simulink library "lib_inverse_clarke_transform"  (R2023a)
settings: Solver=VariableStepAuto  StartTime=0.0  StopTime=10.0  RelTol=1e-3
settings Model: Creator=cav2ofo  LastModifiedBy=lenovo
settings OptimizationCC: ReuseModelBlockBuffer=off

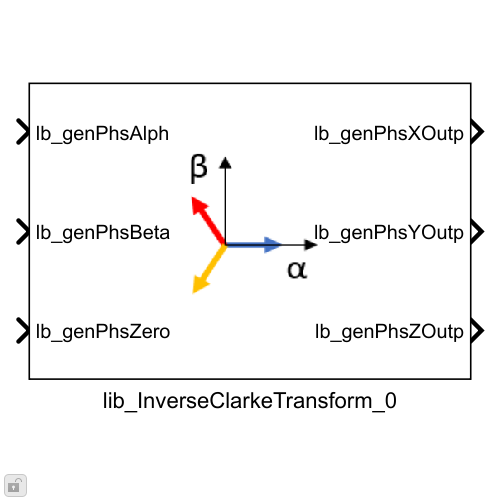
[thumbnail: Simulink's stored preview of the top-level diagram]
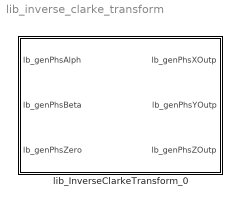
== system lib_inverse_clarke_transform ==
  lib_InverseClarkeTransform_0 : Subsystem  VariantControl=ClarkTransf_MIL_flo  mask{lb_parSymMot=off}
      mask prompts: lb_parSymMot "Asymmetric motor"
      mask DialogControl DescGroupVar Prompt: Inverse Clarke Transform
      mask DialogControl DescTextVar Prompt: VHIT Control Library
      mask DialogControl clarkeDesc Prompt: This block performs Inverse Clarke transform on the input signals. You can choose the computation logic either for symmetric or asymmetric motor type. For symmetric motor type the lb_genPhsZero is zero.
      mask DialogControl blockParam Prompt: Block Parameters
      mask DialogControl Control2 Prompt: By default the computation for symmetric motor is performed. Tick the following check box for asymmetric motor type.
      mask Display: image('ClarkTransf.png'); % Use "Edit Image" on toolstrip to change.

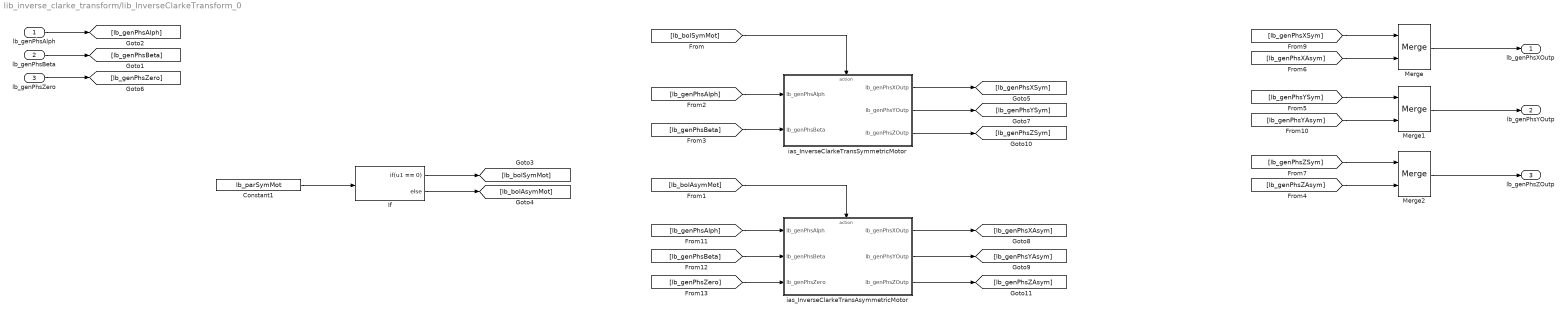
== system lib_inverse_clarke_transform/lib_InverseClarkeTransform_0 ==
  lb_genPhsAlph : Inport
  lb_genPhsBeta : Inport  Port=2
  lb_genPhsZero : Inport  Port=3
  Constant1 : Constant  Value=lb_parSymMot  OutDataTypeStr=boolean
  If : If  IfExpression=u1 == 0
  Merge : Merge
  Merge1 : Merge
  Merge2 : Merge
  ias_InverseClarkeTransAsymmetricMotor : Subsystem  TreatAsAtomicUnit=on
  ias_InverseClarkeTransSymmetricMotor : Subsystem  TreatAsAtomicUnit=on
  lb_genPhsXOutp : Outport  VectorParamsAs1DForOutWhenUnconnected=off
  lb_genPhsYOutp : Outport  Port=2  VectorParamsAs1DForOutWhenUnconnected=off
  lb_genPhsZOutp : Outport  Port=3  VectorParamsAs1DForOutWhenUnconnected=off
  wires:
  [lb_genPhsBeta] -> ias_InverseClarkeTransAsymmetricMotor/2(lb_genPhsBeta)
  If/1 -> [lb_bolSymMot]
  If/2 -> [lb_bolAsymMot]
  Merge2/1 -> lb_genPhsZOutp/1
  [lb_genPhsZSym] -> Merge2/1
  [lb_genPhsZAsym] -> Merge2/2
  ias_InverseClarkeTransAsymmetricMotor/3(lb_genPhsZOutp) -> [lb_genPhsZAsym]
  ias_InverseClarkeTransSymmetricMotor/3(lb_genPhsZOutp) -> [lb_genPhsZSym]
  [lb_genPhsZero] -> ias_InverseClarkeTransAsymmetricMotor/3(lb_genPhsZero)
  [lb_genPhsAlph] -> ias_InverseClarkeTransAsymmetricMotor/1(lb_genPhsAlph)
  lb_genPhsZero/1 -> [lb_genPhsZero]
  lb_genPhsBeta/1 -> [lb_genPhsBeta]
  lb_genPhsAlph/1 -> [lb_genPhsAlph]
  Merge/1 -> lb_genPhsXOutp/1
  Merge1/1 -> lb_genPhsYOutp/1
  [lb_genPhsYSym] -> Merge1/1
  [lb_genPhsYAsym] -> Merge1/2
  [lb_genPhsXAsym] -> Merge/2
  [lb_genPhsXSym] -> Merge/1
  ias_InverseClarkeTransAsymmetricMotor/2(lb_genPhsYOutp) -> [lb_genPhsYAsym]
  ias_InverseClarkeTransAsymmetricMotor/1(lb_genPhsXOutp) -> [lb_genPhsXAsym]
  ias_InverseClarkeTransSymmetricMotor/2(lb_genPhsYOutp) -> [lb_genPhsYSym]
  ias_InverseClarkeTransSymmetricMotor/1(lb_genPhsXOutp) -> [lb_genPhsXSym]
  [lb_genPhsBeta] -> ias_InverseClarkeTransSymmetricMotor/2(lb_genPhsBeta)
  [lb_genPhsAlph] -> ias_InverseClarkeTransSymmetricMotor/1(lb_genPhsAlph)
  [lb_bolAsymMot] -> ias_InverseClarkeTransAsymmetricMotor/Action
  [lb_bolSymMot] -> ias_InverseClarkeTransSymmetricMotor/Action
  Constant1/1 -> If/1

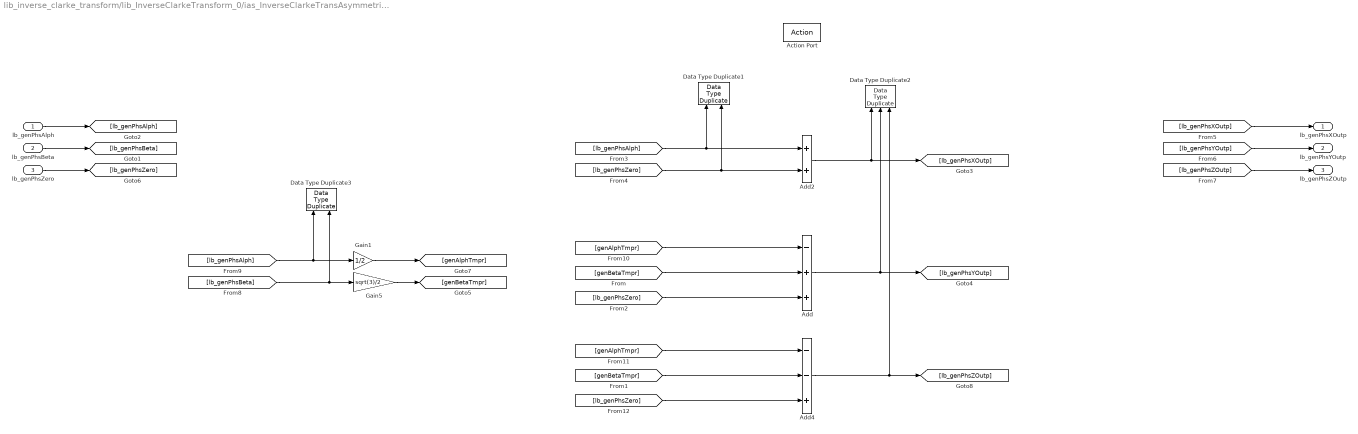
== system lib_inverse_clarke_transform/lib_InverseClarkeTransform_0/ias_InverseClarkeTransAsymmetricMotor ==
  lb_genPhsAlph : Inport
  lb_genPhsBeta : Inport  Port=2
  lb_genPhsZero : Inport  Port=3
  Action Port : ActionPort
  Add : Sum  Inputs=-++  OutDataTypeStr=Inherit: Inherit via back propagation  InputSameDT=on  SaturateOnIntegerOverflow=on
  Add2 : Sum  OutDataTypeStr=Inherit: Inherit via back propagation  InputSameDT=on  SaturateOnIntegerOverflow=on
  Add4 : Sum  Inputs=--+  OutDataTypeStr=Inherit: Inherit via back propagation  InputSameDT=on  SaturateOnIntegerOverflow=on
  Data Type Duplicate1 : DataTypeDuplicate
  Data Type Duplicate2 : DataTypeDuplicate  NumInputPorts=3
  Data Type Duplicate3 : DataTypeDuplicate
  Gain1 : Gain  Gain=1/2  OutDataTypeStr=Inherit: Inherit via back propagation
  Gain5 : Gain  Gain=sqrt(3)/2  ParamDataTypeStr=Inherit: Inherit from 'Gain'  OutDataTypeStr=Inherit: Inherit via back propagation
  lb_genPhsXOutp : Outport  VectorParamsAs1DForOutWhenUnconnected=off
  lb_genPhsYOutp : Outport  Port=2  VectorParamsAs1DForOutWhenUnconnected=off
  lb_genPhsZOutp : Outport  Port=3  VectorParamsAs1DForOutWhenUnconnected=off
  wires:
  [lb_genPhsZero] -> Add4/3
  [genBetaTmpr] -> Add4/2
  Add4/1 -> Data Type Duplicate2/3, [lb_genPhsZOutp]
  [genAlphTmpr] -> Add4/1
  Gain5/1 -> [genBetaTmpr]
  [lb_genPhsAlph] -> Gain1/1, Data Type Duplicate3/1
  [lb_genPhsBeta] -> Gain5/1, Data Type Duplicate3/2
  Gain1/1 -> [genAlphTmpr]
  [genAlphTmpr] -> Add/1
  [lb_genPhsZOutp] -> lb_genPhsZOutp/1
  [lb_genPhsYOutp] -> lb_genPhsYOutp/1
  [lb_genPhsXOutp] -> lb_genPhsXOutp/1
  lb_genPhsAlph/1 -> [lb_genPhsAlph]
  lb_genPhsBeta/1 -> [lb_genPhsBeta]
  lb_genPhsZero/1 -> [lb_genPhsZero]
  [lb_genPhsAlph] -> Add2/1, Data Type Duplicate1/1
  [genBetaTmpr] -> Add/2
  [lb_genPhsZero] -> Add2/2, Data Type Duplicate1/2
  [lb_genPhsZero] -> Add/3
  Add2/1 -> [lb_genPhsXOutp], Data Type Duplicate2/1
  Add/1 -> [lb_genPhsYOutp], Data Type Duplicate2/2

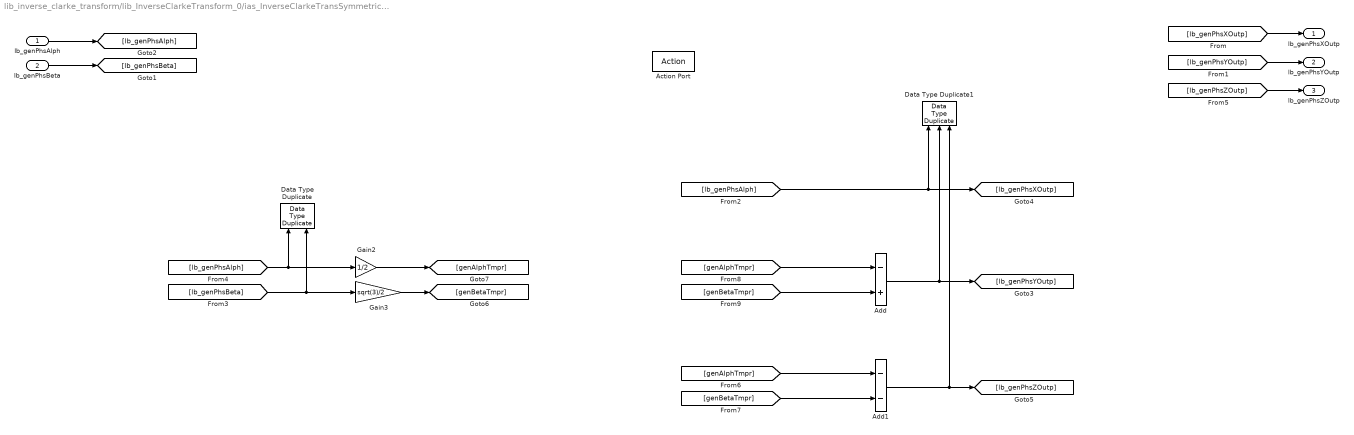
== system lib_inverse_clarke_transform/lib_InverseClarkeTransform_0/ias_InverseClarkeTransSymmetricMotor ==
  lb_genPhsAlph : Inport
  lb_genPhsBeta : Inport  Port=2
  Action Port : ActionPort
  Add : Sum  Inputs=-+  OutDataTypeStr=Inherit: Inherit via back propagation
  Add1 : Sum  Inputs=--  OutDataTypeStr=Inherit: Inherit via back propagation
  Data Type Duplicate : DataTypeDuplicate
  Data Type Duplicate1 : DataTypeDuplicate  NumInputPorts=3
  Gain2 : Gain  Gain=1/2  OutDataTypeStr=Inherit: Inherit via back propagation
  Gain3 : Gain  Gain=sqrt(3)/2  ParamDataTypeStr=Inherit: Inherit from 'Gain'  OutDataTypeStr=Inherit: Inherit via back propagation
  lb_genPhsXOutp : Outport  VectorParamsAs1DForOutWhenUnconnected=off
  lb_genPhsYOutp : Outport  Port=2  VectorParamsAs1DForOutWhenUnconnected=off
  lb_genPhsZOutp : Outport  Port=3  VectorParamsAs1DForOutWhenUnconnected=off
  wires:
  [genAlphTmpr] -> Add/1
  [genBetaTmpr] -> Add/2
  Add1/1 -> Data Type Duplicate1/3, [lb_genPhsZOutp]
  [genBetaTmpr] -> Add1/2
  [genAlphTmpr] -> Add1/1
  Gain2/1 -> [genAlphTmpr]
  [lb_genPhsZOutp] -> lb_genPhsZOutp/1
  [lb_genPhsAlph] -> [lb_genPhsXOutp], Data Type Duplicate1/1
  [lb_genPhsAlph] -> Data Type Duplicate/1, Gain2/1
  Gain3/1 -> [genBetaTmpr]
  lb_genPhsBeta/1 -> [lb_genPhsBeta]
  lb_genPhsAlph/1 -> [lb_genPhsAlph]
  [lb_genPhsYOutp] -> lb_genPhsYOutp/1
  [lb_genPhsXOutp] -> lb_genPhsXOutp/1
  Add/1 -> Data Type Duplicate1/2, [lb_genPhsYOutp]
  [lb_genPhsBeta] -> Gain3/1, Data Type Duplicate/2
